simulink model "ev3Bike"  (R2018a)
settings: Solver=FixedStepAuto  StartTime=0.0  StopTime=10.0  RelTol=1e-3  EnableMultiTasking=on
undefined symbols (not defined in the file or in its folder): DiscIntNeverNeededParam, Lean, LeanDot, Steer, SteerDt, Vel
libraries: legoev3lib x10, simulink x4
settings Model: ExtModeTrigDuration=2  Creator=Philip  LastModifiedBy=Philip
settings SolverCC: PositivePriorityOrder=on  AutoInsertRateTranBlk=on
settings OptimizationCC: EnhancedBackFolding=on  PassReuseOutputArgsThreshold=0  MaxStackSize=64  OptimizeBlockOrder=speed  DifferentSizesBufferReuse=on  OptimizationCustomize=off
settings DebuggingCC: ParameterTunabilityLossMsg=error
settings HardwareCC: ProdBitPerPointer=32  ProdBitPerSizeT=32  ProdBitPerPtrDiffT=32  ProdLargestAtomicInteger=Long  ProdWordSize=32  ProdHWDeviceType=ARM Compatible->ARM 9  UseEmbeddedCoderFeatures=off  UseSimulinkCoderFeatures=off
settings SFSimCC: MATLABDynamicMemAlloc=off
settings RTWCC: SystemTargetFile=ert.tlc  HardwareBoard=LEGO MINDSTORMS EV3  TLCOptions="-aInlineSetEventsForThisBaseRateFcn=TLC_FALSE -aSuppressMultiTaskScheduler=TLC_FALSE  -aRateBasedStepFcn=0"  TemplateMakefile=ert_default_tmf  GenerateReport=on  Toolchain=Sourcery G++ Lite v2009q3  LaunchReport=on
settings CodeAppCC: ForceParamTrailComments=on  OperatorAnnotations=on
settings ERTTargetCC: ERTCustomFileBanners=off  SupportContinuousTime=on  SupportNonInlinedSFcns=on  RemoveResetFunc=off  SupportVariableSizeSignals=on  ModelStepFunctionPrototypeControlCompliant=off

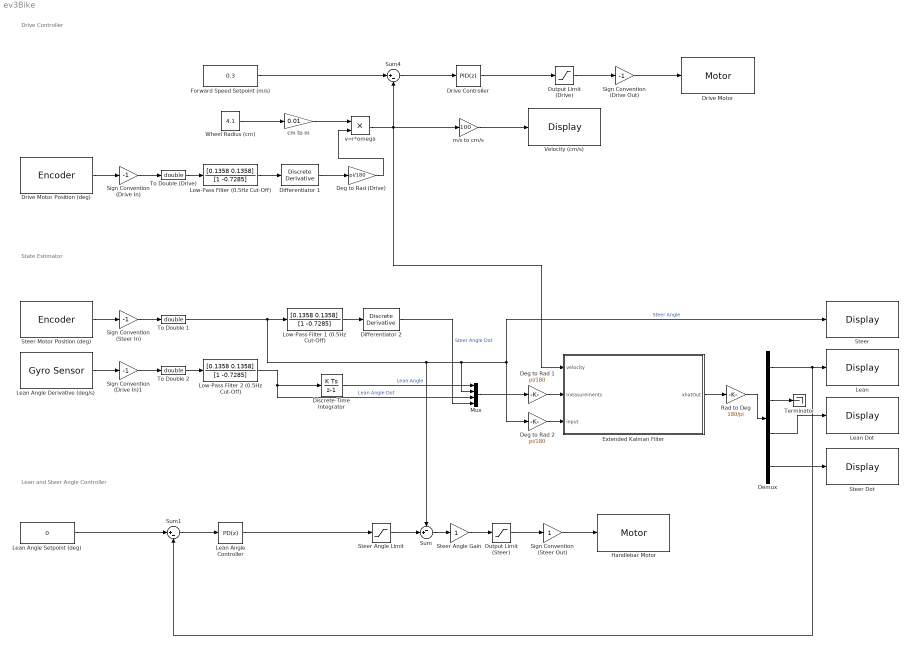
== system ev3Bike ==
  note: Drive Controller
  note: State Estimator
  note: Lean and Steer Angle Controller
  Deg to Rad (Drive) : Gain  Gain=pi/180
  Deg to Rad 1 : Gain  Gain=pi/180
  Deg to Rad 2 : Gain  Gain=pi/180
  Demux : Demux
  Differentiator 1 : simulink/Discrete/Discrete Derivative  gainval=1.0  ICPrevScaledInput=0.0  OutMin=[]  OutMax=[]  OutDataType=fixdt(1, 16)  OutScaling=2^-10  DoSatur=off
  Differentiator 2 : simulink/Discrete/Discrete Derivative  gainval=1.0  ICPrevScaledInput=0.0  OutMin=[]  OutMax=[]  OutDataType=fixdt(1, 16)  OutScaling=2^-10  DoSatur=off
  Discrete-Time Integrator : DiscreteIntegrator  SampleTime=-1  ICPrevOutput=DiscIntNeverNeededParam  ICPrevScaledInput=DiscIntNeverNeededParam
  Drive Controller : simulink/Continuous/PID Controller  Controller=PID  TimeDomain=Discrete-time  SampleTime=-1  IntegratorMethod=Backward Euler  FilterMethod=Forward Euler  Form=Parallel  UseFilter=off  ControllerParametersSource=internal  P=800  I=600  D=100  N=100  InitialConditionSource=internal  InitialConditionForIntegrator=0  InitialConditionForFilter=0  ExternalReset=none  LimitOutput=on  UpperSaturationLimit=100  LowerSaturationLimit=0  LinearizeAsGain=off  AntiWindupMode=back-calculation  Kb=1  TrackingMode=off  Kt=1  PParamMin=[]  PParamMax=[]  IParamMin=[]  IParamMax=[]  DParamMin=[]  DParamMax=[]  NParamMin=[]  NParamMax=[]  KbParamMin=[]  KbParamMax=[]  KtParamMin=[]  KtParamMax=[]  POutMin=[]  POutMax=[]  IOutMin=[]  IOutMax=[]  DOutMin=[]  DOutMax=[]  NOutMin=[]  NOutMax=[]  KbOutMin=[]  KbOutMax=[]  KtOutMin=[]  KtOutMax=[]  IntegratorOutMin=[]  IntegratorOutMax=[]  FilterOutMin=[]  FilterOutMax=[]  SumOutMin=[]  SumOutMax=[]  SumI1OutMin=[]  SumI1OutMax=[]  SumI2OutMin=[]  SumI2OutMax=[]  SumI3OutMin=[]  SumI3OutMax=[]  SumDOutMin=[]  SumDOutMax=[]  SaturationOutMin=[]  SaturationOutMax=[]  IntegratorContinuousStateAttributes=''  IntegratorStateMustResolveToSignalObject=off  IntegratorRTWStateStorageClass=Auto  FilterContinuousStateAttributes=''  FilterStateMustResolveToSignalObject=off  FilterRTWStateStorageClass=Auto  DifferentiatorICPrevScaledInput=0  DifferentiatorOutMin=[]  DifferentiatorOutMax=[]  FilterDiffOutCoefMin=[]  FilterDiffOutCoefMax=[]  SumDenOutMin=[]  SumDenOutMax=[]  SumNumOutMin=[]  SumNumOutMax=[]  ReciprocalOutMin=[]  ReciprocalOutMax=[]  DivideOutMin=[]  DivideOutMax=[]  TunerSelectOption=Transfer Function Based (PID Tuner App)
  Drive Motor : legoev3lib/Motor  sportNumber=B  sstopAction=Brake
  Drive Motor Position (deg) : legoev3lib/Encoder  portNumber=B  opMode=No reset  sampleTime=0.01
      settings: SourceProductName=Simulink Support Package for LEGO MINDSTORMS EV3 Hardware  SourceProductBaseCode=LEGOEV3
  Extended Kalman Filter : MATLAB Function  TreatAsAtomicUnit=on
  Forward Speed Setpoint (m/s) : Constant  Value=0.3
  Handlebar Motor : legoev3lib/Motor  sportNumber=A  sstopAction=Brake
  Lean : legoev3lib/Display  slcdStr=Lean:  slcdLine=2  slcdFormat=Decimal
      settings: SourceProductName=Simulink Support Package for LEGO MINDSTORMS EV3 Hardware  SourceProductBaseCode=LEGOEV3
  Lean Angle Controller : simulink/Continuous/PID Controller  Controller=PD  TimeDomain=Discrete-time  SampleTime=-1  IntegratorMethod=Backward Euler  FilterMethod=Forward Euler  Form=Parallel  UseFilter=off  ControllerParametersSource=internal  P=1  I=600  D=0.5  N=100  InitialConditionSource=internal  InitialConditionForIntegrator=0  InitialConditionForFilter=0  ExternalReset=none  LimitOutput=on  UpperSaturationLimit=100  LowerSaturationLimit=0  LinearizeAsGain=off  AntiWindupMode=back-calculation  Kb=1  TrackingMode=off  Kt=1  PParamMin=[]  PParamMax=[]  IParamMin=[]  IParamMax=[]  DParamMin=[]  DParamMax=[]  NParamMin=[]  NParamMax=[]  KbParamMin=[]  KbParamMax=[]  KtParamMin=[]  KtParamMax=[]  POutMin=[]  POutMax=[]  IOutMin=[]  IOutMax=[]  DOutMin=[]  DOutMax=[]  NOutMin=[]  NOutMax=[]  KbOutMin=[]  KbOutMax=[]  KtOutMin=[]  KtOutMax=[]  IntegratorOutMin=[]  IntegratorOutMax=[]  FilterOutMin=[]  FilterOutMax=[]  SumOutMin=[]  SumOutMax=[]  SumI1OutMin=[]  SumI1OutMax=[]  SumI2OutMin=[]  SumI2OutMax=[]  SumI3OutMin=[]  SumI3OutMax=[]  SumDOutMin=[]  SumDOutMax=[]  SaturationOutMin=[]  SaturationOutMax=[]  IntegratorContinuousStateAttributes=''  IntegratorStateMustResolveToSignalObject=off  IntegratorRTWStateStorageClass=Auto  FilterContinuousStateAttributes=''  FilterStateMustResolveToSignalObject=off  FilterRTWStateStorageClass=Auto  DifferentiatorICPrevScaledInput=0  DifferentiatorOutMin=[]  DifferentiatorOutMax=[]  FilterDiffOutCoefMin=[]  FilterDiffOutCoefMax=[]  SumDenOutMin=[]  SumDenOutMax=[]  SumNumOutMin=[]  SumNumOutMax=[]  ReciprocalOutMin=[]  ReciprocalOutMax=[]  DivideOutMin=[]  DivideOutMax=[]  TunerSelectOption=Transfer Function Based (PID Tuner App)
  Lean Angle Derivative (deg/s) : legoev3lib/Gyro Sensor  portNumber=1  sampleTime=0.01
      settings: SourceProductName=Simulink Support Package for LEGO MINDSTORMS EV3 Hardware  SourceProductBaseCode=LEGOEV3
  Lean Angle Setpoint (deg) : Constant  Value=0
  Lean Dot : legoev3lib/Display  slcdStr=LeanDot:  slcdLine=4  slcdFormat=Decimal
      settings: SourceProductName=Simulink Support Package for LEGO MINDSTORMS EV3 Hardware  SourceProductBaseCode=LEGOEV3
  Low-Pass Filter (0.5Hz Cut-Off) : DiscreteFilter  Numerator=[0.1358 0.1358]  Denominator=[1 -0.7285]
  Low-Pass Filter 1 (0.5Hz Cut-Off) : DiscreteFilter  Numerator=[0.1358 0.1358]  Denominator=[1 -0.7285]
  Low-Pass Filter 2 (0.5Hz Cut-Off) : DiscreteFilter  Numerator=[0.1358 0.1358]  Denominator=[1 -0.7285]
  Mux : Mux
  Output Limit (Steer) : Saturate  UpperLimit=100  LowerLimit=-100
  Output Limit (Drive) : Saturate  UpperLimit=100  LowerLimit=-100
  Rad to Deg : Gain  Gain=180/pi
  Sign Convention (Drive In) : Gain  Gain=-1
  Sign Convention (Drive In)1 : Gain  Gain=-1
  Sign Convention (Drive Out) : Gain  Gain=-1
  Sign Convention (Steer In) : Gain  Gain=-1
  Sign Convention (Steer Out) : Gain
  Steer : legoev3lib/Display  slcdStr=Steer:  slcdLine=3  slcdFormat=Decimal
      settings: SourceProductName=Simulink Support Package for LEGO MINDSTORMS EV3 Hardware  SourceProductBaseCode=LEGOEV3
  Steer Angle Gain : Gain
  Steer Angle Limit : Saturate  UpperLimit=45  LowerLimit=-45
  Steer Dot : legoev3lib/Display  slcdStr=SteerDt:  slcdLine=5  slcdFormat=Decimal
      settings: SourceProductName=Simulink Support Package for LEGO MINDSTORMS EV3 Hardware  SourceProductBaseCode=LEGOEV3
  Steer Motor Position (deg) : legoev3lib/Encoder  portNumber=A  opMode=No reset  sampleTime=0.01
      settings: SourceProductName=Simulink Support Package for LEGO MINDSTORMS EV3 Hardware  SourceProductBaseCode=LEGOEV3
  Sum : Sum  Inputs=-+|
  Sum1 : Sum  Inputs=|+-
  Sum4 : Sum  Inputs=|+-
  Terminator : Terminator
  To Double (Drive) : DataTypeConversion  OutDataTypeStr=double
  To Double 1 : DataTypeConversion  OutDataTypeStr=double
  To Double 2 : DataTypeConversion  OutDataTypeStr=double
  Velocity (cm/s) : legoev3lib/Display  slcdStr=Vel:  slcdLine=1  slcdFormat=Decimal
      settings: SourceProductName=Simulink Support Package for LEGO MINDSTORMS EV3 Hardware  SourceProductBaseCode=LEGOEV3
  Wheel Radius (cm) : Constant  Value=4.1
  cm to m : Gain  Gain=0.01
  m/s to cm/s : Gain  Gain=100
  v=r*omega : Product
  wires:
  Forward Speed Setpoint (m/s)/1 -> Sum4/1
  v=r*omega/1 -> Extended Kalman Filter/1(velocity), Sum4/2, m/s to cm/s/1
  Sum4/1 -> Drive Controller/1
  Wheel Radius (cm)/1 -> cm to m/1
  cm to m/1 -> v=r*omega/1
  Output Limit (Drive)/1 -> Sign Convention (Drive Out)/1
  Sign Convention (Drive Out)/1 -> Drive Motor/1
  Sign Convention (Drive In)/1 -> To Double (Drive)/1
  To Double (Drive)/1 -> Low-Pass Filter (0.5Hz Cut-Off)/1
  Low-Pass Filter (0.5Hz Cut-Off)/1 -> Differentiator 1/1
  Differentiator 1/1 -> Deg to Rad (Drive)/1
  Deg to Rad (Drive)/1 -> v=r*omega/2
  m/s to cm/s/1 -> Velocity (cm/s)/1
  Drive Controller/1 -> Output Limit (Drive)/1
  Drive Motor Position (deg)/1 -> Sign Convention (Drive In)/1
  Deg to Rad 2/1 -> Extended Kalman Filter/3(input)
  To Double 1/1 -> Low-Pass Filter 1 (0.5Hz Cut-Off)/1, Sum/1, Steer/1, Deg to Rad 2/1, Mux/2  "Steer Angle"
  Sign Convention (Drive In)1/1 -> To Double 2/1
  Lean Angle Derivative (deg/s)/1 -> Sign Convention (Drive In)1/1
  Deg to Rad 1/1 -> Extended Kalman Filter/2(measurements)
  Mux/1 -> Deg to Rad 1/1
  Steer Motor Position (deg)/1 -> Sign Convention (Steer In)/1
  Sign Convention (Steer In)/1 -> To Double 1/1
  Low-Pass Filter 1 (0.5Hz Cut-Off)/1 -> Differentiator 2/1
  Differentiator 2/1 -> Mux/4  "Steer Angle Dot"
  Discrete-Time Integrator/1 -> Mux/1  "Lean Angle"
  Demux/1 -> Sum1/2, Lean/1
  Extended Kalman Filter/1(xhatOut) -> Rad to Deg/1
  Rad to Deg/1 -> Demux/1
  Demux/3 -> Lean Dot/1
  Demux/4 -> Steer Dot/1
  To Double 2/1 -> Low-Pass Filter 2 (0.5Hz Cut-Off)/1
  Low-Pass Filter 2 (0.5Hz Cut-Off)/1 -> Mux/3, Discrete-Time Integrator/1  "Lean Angle Dot"
  Demux/2 -> Terminator/1
  Lean Angle Setpoint (deg)/1 -> Sum1/1
  Sum1/1 -> Lean Angle Controller/1
  Lean Angle Controller/1 -> Steer Angle Limit/1
  Sign Convention (Steer Out)/1 -> Handlebar Motor/1
  Steer Angle Limit/1 -> Sum/2
  Output Limit (Steer)/1 -> Sign Convention (Steer Out)/1
  Sum/1 -> Steer Angle Gain/1
  Steer Angle Gain/1 -> Output Limit (Steer)/1

== matlab function ev3Bike/Extended Kalman Filter ==
  data: velocity input; measurements input; xhatOut output; input input
function xhatOut = ExtKalman(velocity, measurements, input)

    % States: x = [phi delta phidot deltadot]

    persistent P xhat Q R
    
    if isempty(P)
       
        xhat = [0; 0; 0; 0];
        P = zeros(4);
        Q = diag([0.1 0.1 0.01 0.01]); % Process noise
        R = diag([1 0.01 0.1 0.1]); % Measurement nosie
        
    end
    
    % Jacobians
    A = [0, 0, 1, 0; ...
         0, 0, 0, 1; ...
         194, -1.47 - 80.5*velocity*velocity, -velocity, -11.9*velocity; ...
         15.1, 229 - 20*velocity*velocity, 20.9*velocity, -8.24*velocity];

    B = [0; 1; 0; 0];
     
    C = diag([1 1 1 1]);

    xhat = A * xhat + B * input;
    P = A * P * A' + Q;
    
    K = P * C' * (C * P * C' + R)^-1;
    
    resid = measurements - C * xhat;
    
    xhat = xhat + K * resid;
    
    P = (eye(4) - K * C) * P;
    
    xhatOut = xhat;
    
end
